simulink model "bus_expand_blk"  (R2019a)
settings: Solver=VariableStepAuto  StartTime=0.0  StopTime=10.0  RelTol=1e-3
libraries: xbsIndex_r4 x7
settings Model: Creator=Ross Donnachie  LastModifiedBy=Ross Donnachie

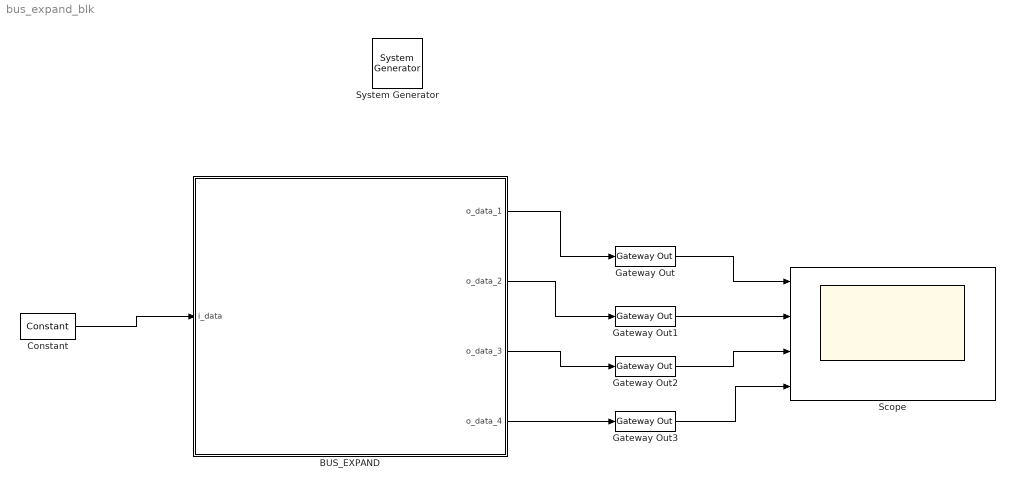
== system bus_expand_blk ==
  " System Generator" : xbsIndex_r4/ System Generator  Tag=genX  xilinxfamily=kintex7  part=xc7k325t  speed=-3  package=fbg676  synthesis_tool=Vivado  clock_wrapper=Clock Enables  directory=./netlist  proj_type=Vivado  Synth_file=Vivado Synthesis Defaults  Impl_file=Vivado Implementation Defaults  testbench=off  simulink_period=1  sysclk_period=10  dcm_input_clock_period=10  incr_netlist=off  trim_vbits=Everywhere in SubSystem  dbl_ovrd=According to Block Masks  core_generation=According to Block Masks  run_coregen=off  deprecated_control=off  eval_field=0  block_type=sysgen
  BUS_EXPAND : Subsystem  mask{bit_selections=1,2,3,2, radix_points=0,0,1,0, types=2,1,1,0}
      mask prompts: bit_selections "Bit-widths of each division:"; radix_points "Radix-position of each division:"; types "Output type of each division (ufix=0, fix=1, bool=2):"
      mask init:
      | Simulink.Block.eval([gcb, '/bus_expand']);
      | 
      | bus_expand_subsys2bb_knit();
      mask DialogControl DescTextVar Prompt: Expands a 'bus' into bit-selections. The input will be divided into the specified number of outputs with the specified bit-widths. Divisions are made consequetively from the most significant bit.
  Constant : xbsIndex_r4/Constant  const=255  gui_display_data_type=Fixed-point  arith_type=Unsigned  n_bits=8  bin_pt=0  preci_type=Single  exp_width=8  frac_width=24  explicit_period=on  period=1  equ=P=C  opselect=C  inp2=PCIN>>17  opr=+  inp1=P  carry=CIN  dbl_ovrd=off  block_type=constant
  Gateway Out{,1..3} (4 alike) : xbsIndex_r4/Gateway Out  inherit_from_input=on  hdl_port=on  rows=4  columns=1  UseAsDAC=off  DACChannel='1'  interface=None  automatic_assignment=on  address_offset=hex2dec('00')  intf_name=''  intf_description=''  timing_constraint=None  locs_specified=off  LOCs={}  io_standard={}  block_type=gatewayout
  Scope : Scope  NumInputPorts=4
  wires:
  Constant/1 -> BUS_EXPAND/1(i_data)
  Gateway Out/1 -> Scope/1
  Gateway Out1/1 -> Scope/2
  BUS_EXPAND/2(o_data_2) -> Gateway Out1/1
  BUS_EXPAND/1(o_data_1) -> Gateway Out/1
  BUS_EXPAND/3(o_data_3) -> Gateway Out2/1
  BUS_EXPAND/4(o_data_4) -> Gateway Out3/1
  Gateway Out3/1 -> Scope/4
  Gateway Out2/1 -> Scope/3

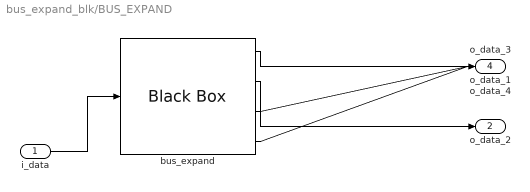
== system bus_expand_blk/BUS_EXPAND ==
  i_data : Inport
  bus_expand : xbsIndex_r4/Black Box  init_code=bus_expand_arbitrary_config  sim_method=ISE Simulator  verbose=on  block_type=blackbox2
  o_data_1 : Outport
  o_data_2 : Outport  Port=2
  o_data_3 : Outport  Port=3
  o_data_4 : Outport  Port=4
  wires:
  i_data/1 -> bus_expand/1
  bus_expand/1 -> o_data_1/1
  bus_expand/2 -> o_data_2/1
  bus_expand/3 -> o_data_3/1
  bus_expand/4 -> o_data_4/1
